simulink model "ACC"  (R2025b)
settings: Solver=FixedStepDiscrete  StartTime=0.0  StopTime=10.0  FixedStep=0.02  RelTol=1e-3
settings Model: DataDictionary=ACC.sldd  Creator=SaiTeja  LastModifiedBy=spadhi
settings OptimizationCC: DefaultParameterBehavior=Inlined  EnhancedBackFolding=on  PassReuseOutputArgsAs=Individual arguments  ZeroExternalMemoryAtStartup=off  ZeroInternalMemoryAtStartup=off  OptimizeBlockOrder=speed  DifferentSizesBufferReuse=on  OptimizationCustomize=off  EfficientTunableParamExpr=on
settings DebuggingCC: ParameterTunabilityLossMsg=error
settings SFSimCC: MATLABDynamicMemAlloc=off
settings RTWCC: SystemTargetFile=ert.tlc  TemplateMakefile=ert_default_tmf  Description=Embedded Coder
settings CodeAppCC: ForceParamTrailComments=on  IgnoreCustomStorageClasses=off  OperatorAnnotations=on  SimulinkDataObjDesc=on  SFDataObjDesc=on  InsertBlockDesc=on
settings ERTTargetCC: ERTCustomFileTemplate=example_file_process.tlc  TargetLangStandard=C99 (ISO)  GenerateSampleERTMain=on

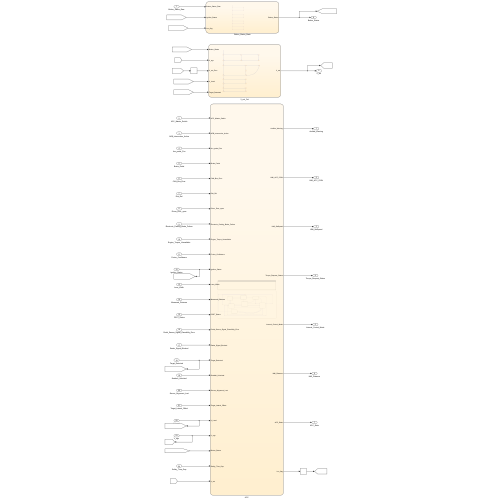
[thumbnail: Simulink's stored preview of the top-level diagram]
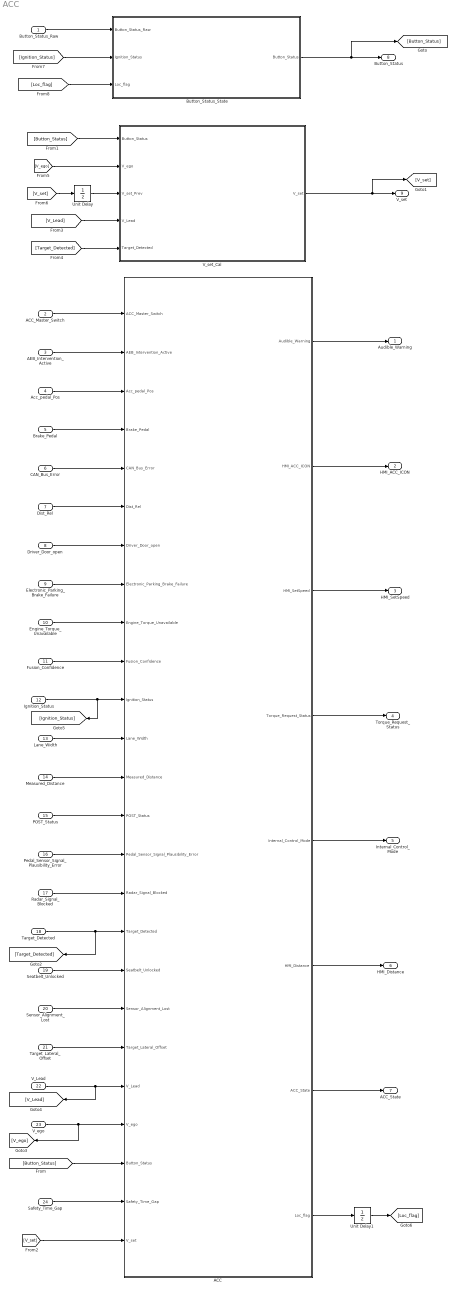
== system ACC ==
  Button_Status_Raw : Inport
  ACC_Master_Switch : Inport  Port=2
  AEB_Intervention_Active : Inport  Port=3
  Acc_pedal_Pos : Inport  Port=4
  Brake_Pedal : Inport  Port=5
  CAN_Bus_Error : Inport  Port=6
  Dist_Rel : Inport  Port=7
  Driver_Door_open : Inport  Port=8
  Electronic_Parking_Brake_Failure : Inport  Port=9
  Engine_Torque_Unavailable : Inport  Port=10
  Fusion_Confidence : Inport  Port=11
  Ignition_Status : Inport  Port=12
  Lane_Width : Inport  Port=13
  Measured_Distance : Inport  Port=14
  POST_Status : Inport  Port=15
  Pedal_Sensor_Signal_Plausibility_Error : Inport  Port=16
  Radar_Signal_Blocked : Inport  Port=17
  Target_Detected : Inport  Port=18
  Seatbelt_Unlocked : Inport  Port=19
  Sensor_Alignment_Lost : Inport  Port=20
  Target_Lateral_Offset : Inport  Port=21
  V_Lead : Inport  Port=22
  V_ego : Inport  Port=23
  Safety_Time_Gap : Inport  Port=24
  ACC : Stateflow chart  TreatAsAtomicUnit=on
  Button_Status_State : Stateflow chart  TreatAsAtomicUnit=on
  Unit Delay : UnitDelay  SampleTime=-1  HasFrameUpgradeWarning=on
  Unit Delay1 : UnitDelay  SampleTime=-1  HasFrameUpgradeWarning=on
  V_set_Cal : Stateflow chart  TreatAsAtomicUnit=on
  Audible_Warning : Outport
  HMI_ACC_ICON : Outport  Port=2
  HMI_SetSpeed : Outport  Port=3
  Torque_Request_Status : Outport  Port=4
  Internal_Control_Mode : Outport  Port=5
  HMI_Distance : Outport  Port=6
  ACC_State : Outport  Port=7
  Button_Status : Outport  Port=8
  V_set : Outport  Port=9
  wires:
  Fusion_Confidence/1 -> ACC/10(Fusion_Confidence)
  Engine_Torque_Unavailable/1 -> ACC/9(Engine_Torque_Unavailable)
  Button_Status_State/1(Button_Status) -> [Button_Status], Button_Status/1
  Button_Status_Raw/1 -> Button_Status_State/1(Button_Status_Raw)
  [Button_Status] -> V_set_Cal/1(Button_Status)
  V_set_Cal/1(V_set) -> V_set/1, [V_set]
  [V_set] -> ACC/25(V_set)
  [V_ego] -> V_set_Cal/2(V_ego)
  ACC_Master_Switch/1 -> ACC/1(ACC_Master_Switch)
  Radar_Signal_Blocked/1 -> ACC/16(Radar_Signal_Blocked)
  CAN_Bus_Error/1 -> ACC/5(CAN_Bus_Error)
  Brake_Pedal/1 -> ACC/4(Brake_Pedal)
  Acc_pedal_Pos/1 -> ACC/3(Acc_pedal_Pos)
  AEB_Intervention_Active/1 -> ACC/2(AEB_Intervention_Active)
  Target_Lateral_Offset/1 -> ACC/20(Target_Lateral_Offset)
  Sensor_Alignment_Lost/1 -> ACC/19(Sensor_Alignment_Lost)
  Seatbelt_Unlocked/1 -> ACC/18(Seatbelt_Unlocked)
  Driver_Door_open/1 -> ACC/7(Driver_Door_open)
  Dist_Rel/1 -> ACC/6(Dist_Rel)
  Electronic_Parking_Brake_Failure/1 -> ACC/8(Electronic_Parking_Brake_Failure)
  Measured_Distance/1 -> ACC/13(Measured_Distance)
  Lane_Width/1 -> ACC/12(Lane_Width)
  Ignition_Status/1 -> [Ignition_Status], ACC/11(Ignition_Status)
  Target_Detected/1 -> [Target_Detected], ACC/17(Target_Detected)
  POST_Status/1 -> ACC/14(POST_Status)
  Pedal_Sensor_Signal_Plausibility_Error/1 -> ACC/15(Pedal_Sensor_Signal_Plausibility_Error)
  V_Lead/1 -> [V_Lead], ACC/21(V_Lead)
  Safety_Time_Gap/1 -> ACC/24(Safety_Time_Gap)
  V_ego/1 -> [V_ego], ACC/22(V_ego)
  [Button_Status] -> ACC/23(Button_Status)
  ACC/3(HMI_SetSpeed) -> HMI_SetSpeed/1
  ACC/1(Audible_Warning) -> Audible_Warning/1
  ACC/2(HMI_ACC_ICON) -> HMI_ACC_ICON/1
  ACC/6(HMI_Distance) -> HMI_Distance/1
  ACC/4(Torque_Request_Status) -> Torque_Request_Status/1
  ACC/5(Internal_Control_Mode) -> Internal_Control_Mode/1
  [V_set] -> Unit Delay/1
  Unit Delay/1 -> V_set_Cal/3(V_set_Prev)
  ACC/7(ACC_State) -> ACC_State/1
  [Target_Detected] -> V_set_Cal/5(Target_Detected)
  [V_Lead] -> V_set_Cal/4(V_Lead)
  [Ignition_Status] -> Button_Status_State/2(Ignition_Status)
  ACC/8(Loc_flag) -> Unit Delay1/1
  [Loc_flag] -> Button_Status_State/3(Loc_flag)
  Unit Delay1/1 -> [Loc_flag]

== stateflow chart ACC/Button_Status_State ==
  (default) -> (junction 29)
  (junction 29) -> (junction 4) [order 1] : [Button_Status_Raw == 1 || Loc_flag]
  (junction 29) -> (junction 8) [order 2]
  (junction 4) -> (junction 6) : {Button_Status = Set}
  (junction 6) -> (junction 8)
  (junction 8) -> (junction 11)
  (junction 11) -> (junction 13) [order 1] : [Button_Status_Raw == 2]
  (junction 11) -> (junction 17) [order 2]
  (junction 13) -> (junction 15) : {Button_Status = Cancel}
  (junction 15) -> (junction 17)
  (junction 17) -> (junction 20)
  (junction 20) -> (junction 32) [order 1] : [Button_Status_Raw == 3]
  (junction 20) -> (junction 35) [order 2]
  (junction 32) -> (junction 34) : {Button_Status = Resume}
  (junction 34) -> (junction 35)
  (junction 35) -> (junction 40)
  (junction 40) -> (junction 39) [order 1] : [(Button_Status_Raw ~= 1 && Button_Status_Raw ~=2 && Button_Status_Raw ~= 3) && (Ignition_Status ~= Ign_Run)]
  (junction 40) -> (junction 42) [order 2]
  (junction 39) -> (junction 41) : {Button_Status = None}
  (junction 41) -> (junction 42)
  data: Button_Status_Raw input; Button_Status output Enum: Dt_Enum_Button_Status_E; Ignition_Status input Enum: Dt_Enum_Ignition_Status_E; Loc_flag input

== stateflow chart ACC/V_set_Cal ==
  (default) -> (junction 2)
  (junction 2) -> (junction 3) [order 1] : [ Button_Status ==Set]
  (junction 3) -> (junction 42) [order 1] : [Target_Detected]
  (junction 2) -> (junction 4) [order 2]
  (junction 3) -> (junction 1) [order 2] : {V_set = V_ego}
  (junction 42) -> (junction 44) : {V_set = V_Lead}
  (junction 1) -> (junction 4)
  (junction 44) -> (junction 1)
  (junction 4) -> (junction 9)
  (junction 9) -> (junction 7) [order 1] : [Button_Status == Resume]
  (junction 7) -> (junction 34) [order 2]
  (junction 34) -> (junction 10) : {V_set = V_set_Prev}
  (junction 9) -> (junction 5) [order 2]
  (junction 7) -> (junction 39) [order 1] : [V_set_Prev ==0 ]
  (junction 39) -> (junction 10) : {V_set = V_ego}
  (junction 10) -> (junction 5)
  (junction 5) -> (junction 53)
  (junction 53) -> (junction 55) [order 1] : [Button_Status == Cancel]
  (junction 53) -> (junction 59) [order 2]
  (junction 55) -> (junction 57) : {V_set = V_set_Prev}
  (junction 57) -> (junction 59)
  (junction 59) -> (junction 62)
  (junction 62) -> (junction 64) [order 1] : [Button_Status == None]
  (junction 62) -> (junction 68) [order 2]
  (junction 64) -> (junction 66) : {V_set = 255}
  (junction 66) -> (junction 68)
  data: Button_Status input Enum: Dt_Enum_Button_Status_E; V_ego input uint8; V_set output uint8; V_set_Prev input uint8; V_Lead input; Target_Detected input

== stateflow chart ACC/ACC ==
  state HMI_Bars = HMI_Distance_Bars [function]
    (junction 523) -> (junction 533) : {HMI_Bars=1}
    (junction 521) -> (junction 523) [order 1] : [Dist_Rel <= 3.5 && Dist_Rel > 2.5]
    (junction 524) -> (junction 533) : {HMI_Bars=2}
    (junction 521) -> (junction 524) [order 2] : [Dist_Rel <= 2.5 && Dist_Rel > 1.5]
    (default) -> (junction 521)
    (junction 525) -> (junction 533) : {HMI_Bars=3}
    (junction 521) -> (junction 525) [order 3] : [Dist_Rel <= 1.5 && Dist_Rel > 0.75]
    (junction 521) -> (junction 526) [order 4] : [Dist_Rel <= 0.75 && Dist_Rel > 0]
    (junction 521) -> (junction 527) [order 5]
    (junction 526) -> (junction 533) : {HMI_Bars=4}
    (junction 527) -> (junction 533) : {HMI_Bars=0}
  state ACC_States [parallel]
    du:
    HMI_Bar = uint8(HMI_Distance_Bars())
    settings: executionOrder=1
    state ACC_Fault
      en:
      ACC_Status = 2;
      ACC_State = ACC_Fault;
      Torque_Request_Status = Fault;
      HMI_ACC_ICON = Red;
      Audible_Warning = Warn_Loud_Chime;
      Internal_Control_Mode = Error;
    state ACC_Off
      en:
      ACC_Status = 0;
      ACC_State = ACC_Off;
      Torque_Request_Status = Disabled;
      HMI_ACC_ICON = Off;
      HMI_SetSpeed = 0;
      Audible_Warning = Warn_None;
      Internal_Control_Mode = Standstill;
    state ACC_Override
      en:
      ACC_Status = 6;
      ACC_State = ACC_Override;
      Torque_Request_Status = Override;
      HMI_ACC_ICON = Blink_Green;
      Audible_Warning = Warn_Chime;%V>Vset for x
      Internal_Control_Mode = Passive;
    state ACC_Active
      en:
      ACC_Status = 3;
      ACC_State = ACC_Active;
      Torque_Request_Status = Longi;
      HMI_ACC_ICON = Green;
      HMI_SetSpeed = V_set;%Current_SetSpeed
      Audible_Warning = Warn_Single_Beep;
      Internal_Control_Mode = Speedctrl;
      ex:
      Loc_flag=false;
    state ACC_Active_Follow
      en:
      ACC_Status = 4;
      ACC_State =  ACC_Active_Follow;
      %Drel Cal
      Torque_Request_Status = Dis_active;
      HMI_ACC_ICON = Green;
      HMI_SetSpeed = V_set;%New_SetSpeed_Target
      Audible_Warning = Warn_None;
      Internal_Control_Mode = Distctrl;
      du:
      HMI_Distance = HMI_Bar;%1-5 Bars
    state ACC_Standby
      en:
      ACC_Status = 1;
      ACC_State = ACC_Standby;
      Torque_Request_Status = Standby;
      HMI_ACC_ICON = White;
      HMI_SetSpeed = V_set;%Prev Speed
      Audible_Warning = Warn_None;
      Internal_Control_Mode = Monitoring;
    state ACC_Stop_Hold
      en:
      ACC_Status = 5;
      ACC_State = ACC_Stop_Hold;
      Torque_Request_Status = Hold_Req;
      HMI_ACC_ICON = Green;
      Audible_Warning = Warn_None;
      Internal_Control_Mode = Standstill;
    (junction 371) -> (junction 378)
    (junction 384) -> (junction 371)
    (junction 378) -> (junction 373)
    (junction 383) -> (junction 373)
    (junction 374) -> (junction 373)
    (junction 386) -> (junction 383)
    (junction 373) -> ACC_Fault
    (junction 380) -> (junction 374)
    (default) -> ACC_Off
    ACC_Override -> (junction 375) [order 2] : [Brake_Pedal == Pedal_Pressed || ...
        | Button_Status == Cancel]
    (junction 375) -> (junction 425)
    ACC_Off -> ACC_Fault [order 2] : [Ignition_Status == Ign_Run &&...
        | ACC_Master_Switch == Switch_On &&...
        | POST_Status == Failed]
    ACC_Active_Follow -> ACC_Override [order 3] : [Acc_pedal_Pos > 15]
    ACC_Override -> ACC_Fault [order 1] : [Pedal_Sensor_Signal_Plausibility_Error == true  ]
    ACC_Fault -> ACC_Off : [Ignition_Status == Ign_Off ||...
        | ACC_Master_Switch == Switch_Off]
    ACC_Active -> ACC_Fault [order 4] : [Radar_Signal_Blocked == true || ...
        | Engine_Torque_Unavailable == true]
    ACC_Active -> ACC_Override [order 1] : [Acc_pedal_Pos > 15]
    ACC_Override -> (junction 556) [order 3] : [Acc_pedal_Pos < 5 ]
    ACC_Off -> ACC_Standby [order 1] : [Ignition_Status == Ign_Run &&...
        | ACC_Master_Switch == Switch_On &&...
        | POST_Status == Success]
    ACC_Standby -> ACC_Off [order 3] : [Ignition_Status == Ign_Off ||...
        | ACC_Master_Switch == Switch_Off]
    (junction 556) -> ACC_Active_Follow [order 1] : [ Target_Detected == true]
    (junction 556) -> ACC_Active [order 2] : [ Target_Detected == false]
    ACC_Active_Follow -> (junction 380) [order 5] : [ ( Fusion_Confidence > 0 && Fusion_Confidence < 40) || AEB_Intervention_Active == true]
    ACC_Standby -> (junction 386) [order 4] : [CAN_Bus_Error == true ||...
        | Sensor_Alignment_Lost == true]
    ACC_Active -> ACC_Standby [order 3] : [Button_Status == Cancel]
    ACC_Active -> ACC_Active_Follow [order 2] : [Target_Detected == true &&...
        |  Measured_Distance < (single(0.278*single(V_ego)*Safety_Time_Gap))]
    (junction 381) -> ACC_Standby
    (junction 408) -> (junction 381)
    ACC_Standby -> ACC_Active [order 1] : [(Button_Status == Set || ...
        | Button_Status == Resume) && ...
        | V_ego >= 30 && ...
        | Brake_Pedal == Pedal_Released && ...
        | Target_Detected == false]
    ACC_Active_Follow -> ACC_Active [order 1] : [Target_Detected == false ||...
        | Target_Lateral_Offset > Lane_Width ||...
        |  Measured_Distance > (single(0.278*single(V_ego)*Safety_Time_Gap)+Dist_Hyst)]/{Loc_flag=true;}
    (junction 382) -> ACC_Standby
    (junction 421) -> (junction 382)
    ACC_Standby -> ACC_Active_Follow [order 2] : [(Button_Status == Set ||...
        | Button_Status == Resume) && ...
        | V_ego >= 30 && ...
        | Brake_Pedal == Pedal_Released && ...
        | Target_Detected == true]
    ACC_Stop_Hold -> ACC_Standby [order 2] : [Driver_Door_open == true || ...
        | Seatbelt_Unlocked == true || ...
        | Brake_Pedal == Pedal_Pressed]
    ACC_Stop_Hold -> ACC_Active_Follow [order 1] : [ V_Lead > 5 && Dist_Rel > 3.5]
    ACC_Active_Follow -> ACC_Stop_Hold [order 2] : [V_ego < 1 && V_Lead == 0 && Dist_Rel < 3.5]
    ACC_Active_Follow -> (junction 397) [order 4] : [Brake_Pedal == Pedal_Pressed || Button_Status == Cancel]
    ACC_Stop_Hold -> (junction 384) [order 3] : [Electronic_Parking_Brake_Failure == true]
    (junction 397) -> (junction 421)
    (junction 425) -> (junction 408)
  data: HMI_Bars function_output; ACC_Master_Switch input Enum: Dt_Enum_ACC_Master_Switch_E; AEB_Intervention_Active input boolean; Acc_pedal_Pos input uint8; Brake_Pedal input Enum: Dt_Enum_Brk_Pedal_E; CAN_Bus_Error input boolean; Dist_Rel input single; Driver_Door_open input boolean; Electronic_Parking_Brake_Failure input boolean; Engine_Torque_Unavailable input boolean; Fusion_Confidence input uint8; Ignition_Status input Enum: Dt_Enum_Ignition_Status_E; Lane_Width input uint16; Measured_Distance input single; POST_Status input Enum: Dt_Enum_POST_Status_E; Pedal_Sensor_Signal_Plausibility_Error input boolean; Radar_Signal_Blocked input boolean; Target_Detected input boolean; Seatbelt_Unlocked input boolean; Sensor_Alignment_Lost input boolean; Target_Lateral_Offset input uint16; V_Lead input uint8; V_ego input uint8; Button_Status input Enum: Dt_Enum_Button_Status_E; Safety_Time_Gap input single; Audible_Warning output Enum: Dt_Enum_Audible_Warning_E; HMI_ACC_ICON output Enum: Dt_Enum_HMI_ACC_ICON_E; HMI_SetSpeed output uint8; Torque_Request_Status output Enum: Dt_Enum_Torque_Request_Status_E; Internal_Control_Mode output Enum: Dt_Enum_Internal_Control_Mode_E; HMI_Distance output uint8; ACC_Status local uint8 =0; V_set input uint8; ACC_State output Enum: Dt_Enum_ACC_State_E; HMI_Bar local uint8; Dist_Hyst constant single =5; Loc_flag output boolean
